simulink model "AB3Auf1simlnk"  (R2024b)
settings: Solver=ode4  StartTime=0.0  StopTime=20  FixedStep=delta  RelTol=1e-3
values from neighbouring files (symbols this model uses):
  A = [0        -(k1+k2)/m1     0            k2/m1;      1        0               0            0;      0        k2/m2           0            -(k2+k3)/m2;      0        0               1            0]    [AB1Auf2.m]    (also in AB1Auf4.m = [ -0.05    -0.003     -0.98      0.2;       -1       -0.75  ; AB2Auf2.m = [-2 1 0; -10 0 -15; 0 1 0]; AB3Auf1.m = [Y_beta/u0 -(1-Y_r/u0); N_beta N_r])
  B = [0 0; 1.7 -0.2; 0.3 -0.6; 0 0]    [AB1Auf4.m]    (also in AB2Auf2.m = [0; -5; 0]; AB3Auf1.m = [Y_del_rud;N_del_rud])
  beta_0 = deg2rad(6)    [AB3Auf1.m]
  C = eye(size(A))    [AB1Auf4.m]    (also in AB2Auf2.m = eye(3,3); AB3Auf1.m)
  D = zeros(size(B))    [AB1Auf4.m]    (also in AB2Auf2.m = zeros(3,1); AB3Auf1.m; AB5Auf1.m = a1 ./ (2 * Omega_0); AB6.m = -real(L(1)) / omega_0)
  r_0 = deg2rad(2)    [AB3Auf1.m]
settings Model: Creator=the_main_notebook  LastModifiedBy=the_main_notebook

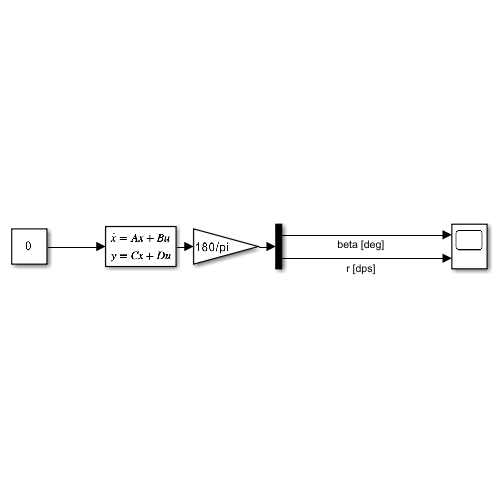
[thumbnail: Simulink's stored preview of the top-level diagram]
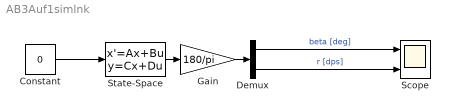
== system AB3Auf1simlnk ==
  Constant : Constant  Value=0
  Demux : Demux  Outputs=2
  Gain : Gain  Gain=180/pi
  Scope : Scope  NumInputPorts=2
  State-Space : StateSpace  A=A  B=B  C=C  D=D  InitialCondition=[beta_0; r_0]
  wires:
  Constant/1 -> State-Space/1
  State-Space/1 -> Gain/1
  Demux/1 -> Scope/1  "beta [deg]"
  Demux/2 -> Scope/2  "r [dps]"
  Gain/1 -> Demux/1
